simulink model "lab_exercice3"  (R2016a)
settings: Solver=FixedStepDiscrete  StartTime=0.0  StopTime=0.1  FixedStep=1/100000  RelTol=1e-3
libraries: dsparch4 x4, dspsrcs4 x1, dspsigops x1
settings Model: Creator=beac2832  LastModifiedBy=beac2832

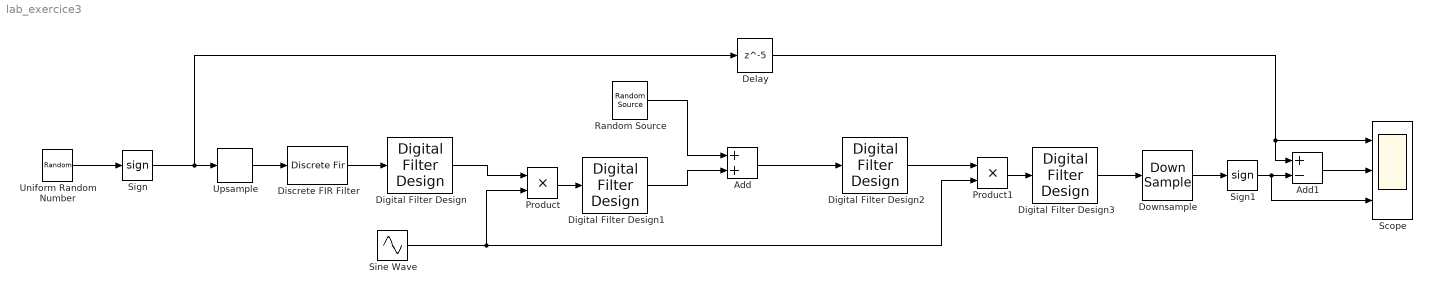
== system lab_exercice3 ==
  Add : Sum
  Add1 : Sum  Inputs=+-
  Delay : Delay  DelayLength=5  InitialCondition=0
  Digital Filter Design{,1..3} (4 alike) : dsparch4/Digital Filter Design  mwdsp_browser_bugfix_var=off
  Discrete FIR Filter : DiscreteFir  Coefficients=ones(1,100)
  Downsample : DownSample  N=100  phase=50  RateOptions=Allow multirate processing
  Product : Product
  Product1 : Product
  Random Source : dspsrcs4/Random Source  SrcType=Gaussian  NormMethod=Ziggurat  CltLength=12  MinVal=0  MaxVal=1  MeanVal=0  VarVal=2  RepMode=Not repeatable  rawSeed=1  IsInherit=on  SampMode=Discrete  SampTime=1  SampFrame=1  DataType=Double  OutComplex=Real  OutputFrames=off
  Scope : Scope  NumInputPorts=3
  Sign : Signum
  Sign1 : Signum
  Sine Wave : Sin  Frequency=10000*2*pi  Phase=pi/2  SampleTime=1/100000
  Uniform Random Number : UniformRandomNumber  SampleTime=1/1000
  Upsample : dspsigops/Upsample  N=100  phase=0  RateOptions=Allow multirate processing  ic=0  mode=Unused parameter value
  wires:
  Uniform Random Number/1 -> Sign/1
  Sign/1 -> Delay/1, Upsample/1
  Upsample/1 -> Discrete FIR Filter/1
  Discrete FIR Filter/1 -> Digital Filter Design/1
  Digital Filter Design/1 -> Product/1
  Sine Wave/1 -> Product1/2, Product/2
  Product/1 -> Digital Filter Design1/1
  Digital Filter Design1/1 -> Add/2
  Add/1 -> Digital Filter Design2/1
  Digital Filter Design2/1 -> Product1/1
  Product1/1 -> Digital Filter Design3/1
  Downsample/1 -> Sign1/1
  Digital Filter Design3/1 -> Downsample/1
  Delay/1 -> Scope/1, Add1/1
  Add1/1 -> Scope/2
  Sign1/1 -> Scope/3, Add1/2
  Random Source/1 -> Add/1
